simulink model "compensate"  (R2018a)
settings: Solver=FixedStepAuto  StartTime=0.0  StopTime=100  FixedStep=0.01  RelTol=1e-3
values from neighbouring files (symbols this model uses):
  a_t = 4    [plot_actuator.m]
  p_limits = [20*pi/180 200]    [plot_actuator.m]    (also in test_allo.m = 20)
libraries: simulink x1
settings Model: Creator=mengc  LastModifiedBy=mengc

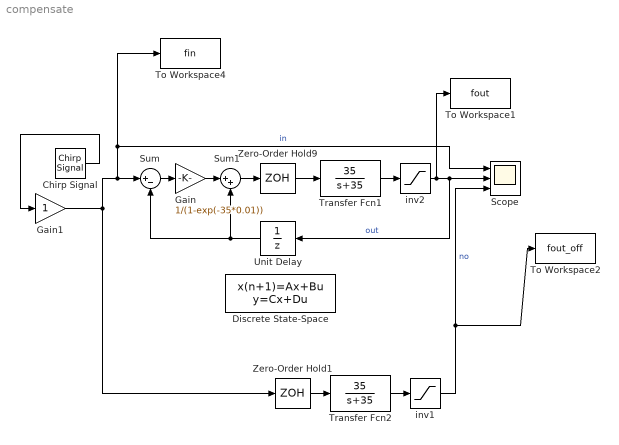
== system compensate ==
  Chirp Signal : simulink/Sources/Chirp Signal  f1=0.1  T=100  f2=2
  Discrete State-Space : DiscreteStateSpace  A=exp(-0.01*a_t)  B=1-exp(-0.01*a_t)  D=0  SampleTime=-1
  Gain : Gain  Gain=1/(1-exp(-35*0.01))
  Gain1 : Gain
  Scope : Scope  NumInputPorts=3
  Sum : Sum  Inputs=|+-
  Sum1 : Sum  Inputs=|++
  To Workspace1 : ToWorkspace  VariableName=fout  SaveFormat=Timeseries  SampleTime=-1
  To Workspace2 : ToWorkspace  VariableName=fout_off  SaveFormat=Timeseries  SampleTime=-1
  To Workspace4 : ToWorkspace  VariableName=fin  SaveFormat=Timeseries  SampleTime=-1
  Transfer Fcn1 : TransferFcn  Numerator=35  Denominator=[1 35]
  Transfer Fcn2 : TransferFcn  Numerator=35  Denominator=[1 35]
  Unit Delay : UnitDelay  SampleTime=-1
  Zero-Order Hold1 : ZeroOrderHold  SampleTime=-1
  Zero-Order Hold9 : ZeroOrderHold  SampleTime=-1
  inv1 : Saturate  UpperLimit=p_limits(2)  LowerLimit=-p_limits(2)
  inv2 : Saturate  UpperLimit=p_limits(2)  LowerLimit=-p_limits(2)
  wires:
  Chirp Signal/1 -> Gain1/1
  Gain1/1 -> Zero-Order Hold1/1, Scope/1, To Workspace4/1, Sum/1  "in"
  Zero-Order Hold9/1 -> Transfer Fcn1/1
  Gain/1 -> Sum1/1
  Sum/1 -> Gain/1
  inv2/1 -> To Workspace1/1, Scope/2, Unit Delay/1  "out"
  Zero-Order Hold1/1 -> Transfer Fcn2/1
  inv1/1 -> Scope/3, To Workspace2/1  "no"
  Unit Delay/1 -> Sum/2, Sum1/2
  Sum1/1 -> Zero-Order Hold9/1
  Transfer Fcn1/1 -> inv2/1
  Transfer Fcn2/1 -> inv1/1
